simulink model "pt8612_dpll_fpga"  (Simulink 5.0)
settings: Solver=ode45  StartTime=0.0  StopTime=10  RelTol=1e-9  AbsTol=1e-12
values from neighbouring files (symbols this model uses):
  alpha = 2^-24    (= 5.96046447754e-08)    [DPLL_init_2.m]    (also in pt8612_dpll_fpga_init.m = -7; pt8612_dpll_fpga_init_2.m = -5)
  beta = 2^-10    (= 0.0009765625)    [DPLL_init_2.m]    (also in pt8612_dpll_fpga_init.m = 5; pt8612_dpll_fpga_init_2.m = 6)
  C = 680e-9    (= 6.8e-07)    [DPLL_init_2.m]    (also in pt8612_analog_pll_init.m = [1 0]; pt8612_analog_pll_init_2.m = [0 1 0]; pt8612_dpll_fpga_init.m; pt8612_dpll_fpga_init_2.m)
  fvcxo = 148.5e6/1.001    (= 148351648.352)    [DPLL_init_2.m]    (also in pt8612_analog_pll_init.m; pt8612_analog_pll_init_2.m; pt8612_dpll_fpga_init.m; pt8612_dpll_fpga_init_2.m = 148500000)
  Kvcxo = 90e-6    (= 9e-05)    [DPLL_init_2.m]    (also in pt8612_analog_pll_init.m; pt8612_analog_pll_init_2.m; pt8612_dpll_fpga_init.m; pt8612_dpll_fpga_init_2.m)
  Mdac = 3/4    (= 0.75)    [DPLL_init_2.m]    (also in pt8612_dpll_fpga_init.m = 1; pt8612_dpll_fpga_init_2.m = 1)
  Nbits = 16    [DPLL_init_2.m]    (also in pt8612_dpll_fpga_init.m; pt8612_dpll_fpga_init_2.m)
  Ndec1 = 91    [DPLL_init_2.m]    (also in pt8612_analog_pll_init.m; pt8612_analog_pll_init_2.m; pt8612_dpll_fpga_init.m = 364)
  Ndec2 = 500    [DPLL_init_2.m]    (also in pt8612_analog_pll_init.m; pt8612_analog_pll_init_2.m; pt8612_dpll_fpga_init.m = 2000)
  R = 1/(wkneeloop*20)/C    (= 4060.30501089)    [DPLL_init_2.m]    (also in pt8612_dpll_fpga_init.m; pt8612_dpll_fpga_init_2.m = 3900)
  Tdac = 4/148.5e6    (= 2.6936026936e-08)    [DPLL_init_2.m]    (also in pt8612_dpll_fpga_init.m)
  Tpll = 1/fpll    (= 3.37037037037e-06)    [DPLL_init_2.m]    (also in pt8612_dpll_fpga_init.m = 1.34814814815e-05)
  Vcc = 3.3    [DPLL_init_2.m]    (also in pt8612_analog_pll_init.m; pt8612_analog_pll_init_2.m; pt8612_dpll_fpga_init.m = 2.5; pt8612_dpll_fpga_init_2.m = 2.5)
  Vvcxo0 = 1.25    [DPLL_init_2.m]    (also in pt8612_analog_pll_init.m; pt8612_analog_pll_init_2.m; pt8612_dpll_fpga_init.m; pt8612_dpll_fpga_init_2.m)
  Vvcxomax = 2.5    [DPLL_init_2.m]    (also in pt8612_analog_pll_init.m; pt8612_analog_pll_init_2.m; pt8612_dpll_fpga_init.m; pt8612_dpll_fpga_init_2.m)
  Vvcxomin = 0    [DPLL_init_2.m]    (also in pt8612_analog_pll_init.m; pt8612_analog_pll_init_2.m; pt8612_dpll_fpga_init.m; pt8612_dpll_fpga_init_2.m)
libraries: simulink x3
settings Model: LastModifiedBy=thh

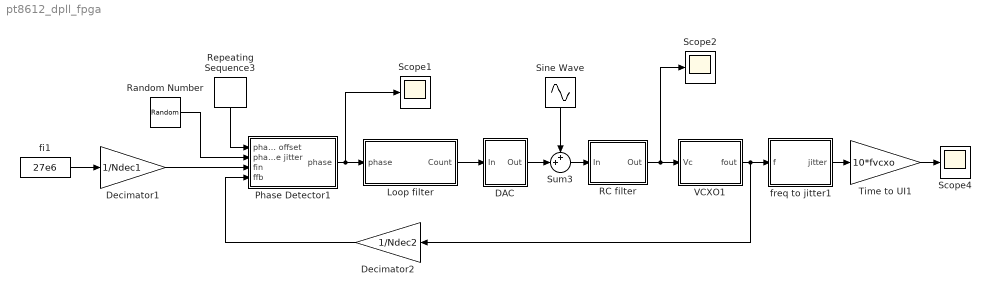
== system pt8612_dpll_fpga ==
  DAC : Subsystem
  Decimator1 : Gain  Gain=1/Ndec1  SaturateOnIntegerOverflow=on
  Decimator2 : Gain  Orientation=left  Gain=1/Ndec2  SaturateOnIntegerOverflow=on
  Loop filter : Subsystem
  Phase Detector1 : Subsystem
  RC filter : Subsystem
  Random Number : RandomNumber  Variance=0  SampleTime=Tpll
  Repeating Sequence3 : simulink/Sources/Repeating Sequence  Orientation=down  rep_seq_t=[0 0.5 0.5 1]*5  rep_seq_y=[0 0 1 1]*5
  Scope1 : Scope
      settings: TimeRange=10  YMin=-250  YMax=5500  SampleInput=on  SampleTime=Tpll
  Scope2 : Scope
      settings: TimeRange=10  YMin=0.22  YMax=0.29  SaveName=ScopeData3  SampleInput=on  SampleTime=1e-4
  Scope4 : Scope
      settings: TimeRange=10  YMin=-3020  YMax=-2977.5  SaveName=ScopeData2  SampleInput=on  SampleTime=1e-4
  Sine Wave : Sin  Orientation=down  Amplitude=0  Frequency=2*pi*25  SampleTime=0
  Sum3 : Sum  Inputs=++|  SaturateOnIntegerOverflow=on
  Time to UI1 : Gain  Gain=10*fvcxo  SaturateOnIntegerOverflow=on
  VCXO1 : Subsystem
  fi1 : Constant  Value=27e6
  freq to jitter1 : Subsystem
  wires:
  freq to jitter1/1(jitter) -> Time to UI1/1
  Time to UI1/1 -> Scope4/1
  Decimator2/1 -> Phase Detector1/4(ffb)
  Phase Detector1/1(phase) -> Loop filter/1(phase), Scope1/1
  Decimator1/1 -> Phase Detector1/3(fin)
  fi1/1 -> Decimator1/1
  RC filter/1(Out) -> VCXO1/1(Vc), Scope2/1
  Repeating Sequence3/1 -> Phase Detector1/1(phase offset)
  Random Number/1 -> Phase Detector1/2(phase jitter)
  DAC/1(Out) -> Sum3/2
  Sum3/1 -> RC filter/1(In)
  VCXO1/1(fout) -> freq to jitter1/1(f), Decimator2/1
  Loop filter/1(Count) -> DAC/1(In)
  Sine Wave/1 -> Sum3/1

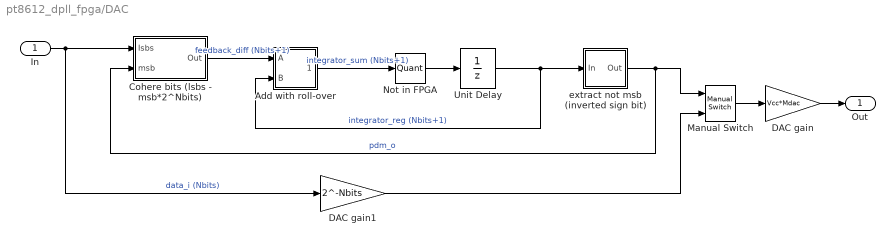
== system pt8612_dpll_fpga/DAC ==
  In : Inport
  Add with roll-over : Subsystem
  Cohere bits (lsbs - msb*2^Nbits) : Subsystem
  DAC gain : Gain  Gain=Vcc*Mdac  SaturateOnIntegerOverflow=on
  DAC gain1 : Gain  Gain=2^-Nbits  SaturateOnIntegerOverflow=on
  Manual Switch : simulink/Signal Routing/Manual Switch  sw=0  action=0
  Not in FPGA : Quantizer  QuantizationInterval=1
  Unit Delay : UnitDelay  SampleTime=Tdac
  extract not msb (inverted sign bit) : Subsystem
  Out : Outport
  wires:
  In/1 -> DAC gain1/1, Cohere bits (lsbs - msb*2^Nbits)/1(Isbs)  "data_i (Nbits)"
  extract not msb (inverted sign bit)/1(Out) -> Cohere bits (lsbs - msb*2^Nbits)/2(msb), Manual Switch/1  "pdm_o"
  Unit Delay/1 -> Add with roll-over/2(B), extract not msb (inverted sign bit)/1(In)  "integrator_reg (Nbits+1)"
  DAC gain/1 -> Out/1
  Not in FPGA/1 -> Unit Delay/1
  Cohere bits (lsbs - msb*2^Nbits)/1(Out) -> Add with roll-over/1(A)  "feedback_diff (Nbits+1)"
  Add with roll-over/1(A+B) -> Not in FPGA/1  "integrator_sum (Nbits+1)"
  DAC gain1/1 -> Manual Switch/2
  Manual Switch/1 -> DAC gain/1

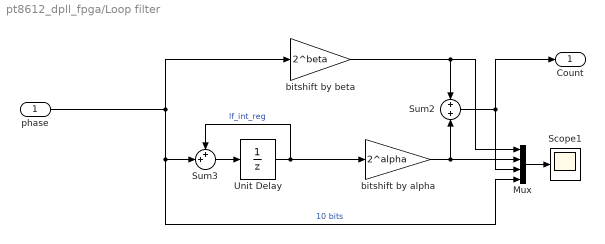
== system pt8612_dpll_fpga/Loop filter ==
  phase : Inport
  Mux : Mux
  Scope1 : Scope
      settings: TimeRange=10  YMin=-500  YMax=9000  SaveName=ScopeData5  Decimation=100  SampleInput=on  SampleTime=Tpll*100
  Sum2 : Sum  SaturateOnIntegerOverflow=on
  Sum3 : Sum  Inputs=++|  SaturateOnIntegerOverflow=on
  Unit Delay : UnitDelay  X0=3.31e4*2^9  SampleTime=Tpll
  bitshift by alpha : Gain  Gain=2^alpha  SaturateOnIntegerOverflow=on
  bitshift by beta : Gain  Gain=2^beta  SaturateOnIntegerOverflow=on
  Count : Outport
  wires:
  phase/1 -> bitshift by beta/1, Mux/4, Sum3/2  "10 bits"
  Sum2/1 -> Count/1, Mux/3
  bitshift by beta/1 -> Sum2/1, Mux/1
  bitshift by alpha/1 -> Sum2/2, Mux/2
  Mux/1 -> Scope1/1
  Unit Delay/1 -> bitshift by alpha/1, Sum3/1  "lf_int_reg"
  Sum3/1 -> Unit Delay/1

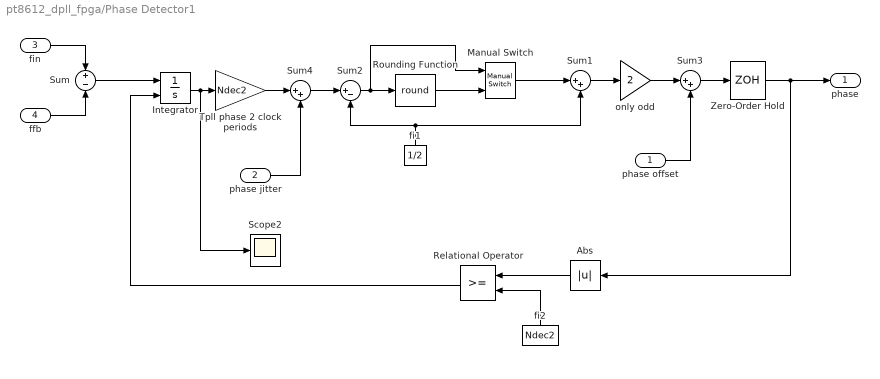
== system pt8612_dpll_fpga/Phase Detector1 ==
  phase offset : Inport
  phase jitter : Inport  Port=2
  fin : Inport  Port=3
  ffb : Inport  Port=4
  Abs : Abs  Orientation=left  SaturateOnIntegerOverflow=on
  Integrator : Integrator  ExternalReset=level
  Manual Switch : simulink/Signal Routing/Manual Switch  sw=0  action=0
  Relational Operator : RelationalOperator  Orientation=left
  Rounding Function : Rounding  Operator=round
  Scope2 : Scope
      settings: TimeRange=10  YMin=1.38778e-017  YMax=0.5  SampleInput=on  SampleTime=1e-4
  Sum : Sum  Inputs=+-  SaturateOnIntegerOverflow=on
  Sum1 : Sum  Inputs=|++  SaturateOnIntegerOverflow=on
  Sum2 : Sum  Inputs=|+-  SaturateOnIntegerOverflow=on
  Sum3 : Sum  Inputs=|++  SaturateOnIntegerOverflow=on
  Sum4 : Sum  Inputs=|++  SaturateOnIntegerOverflow=on
  Tpll phase 2 clock periods : Gain  Gain=Ndec2  SaturateOnIntegerOverflow=on
  Zero-Order Hold : ZeroOrderHold  SampleTime=Tpll
  fi1 : Constant  Orientation=up  Value=1/2
  fi2 : Constant  Orientation=up  Value=Ndec2
  only odd : Gain  Gain=2  SaturateOnIntegerOverflow=on
  phase : Outport
  wires:
  ffb/1 -> Sum/2
  fin/1 -> Sum/1
  Sum/1 -> Integrator/1
  Integrator/1 -> Tpll phase 2 clock periods/1, Scope2/1
  fi1/1 -> Sum1/2, Sum2/2
  Sum2/1 -> Manual Switch/1, Rounding Function/1
  phase offset/1 -> Sum3/2
  Sum3/1 -> Zero-Order Hold/1
  Sum1/1 -> only odd/1
  Manual Switch/1 -> Sum1/1
  Rounding Function/1 -> Manual Switch/2
  phase jitter/1 -> Sum4/2
  Sum4/1 -> Sum2/1
  Tpll phase 2 clock periods/1 -> Sum4/1
  only odd/1 -> Sum3/1
  Abs/1 -> Relational Operator/1
  fi2/1 -> Relational Operator/2
  Relational Operator/1 -> Integrator/2
  Zero-Order Hold/1 -> phase/1, Abs/1

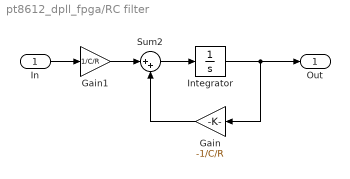
== system pt8612_dpll_fpga/RC filter ==
  In : Inport
  Gain : Gain  Orientation=left  Gain=-1/C/R  SaturateOnIntegerOverflow=on
  Gain1 : Gain  Gain=1/C/R  SaturateOnIntegerOverflow=on
  Integrator : Integrator  InitialCondition=Vvcxo0
  Sum2 : Sum  Inputs=|++  SaturateOnIntegerOverflow=on
  Out : Outport
  wires:
  In/1 -> Gain1/1
  Integrator/1 -> Out/1, Gain/1
  Sum2/1 -> Integrator/1
  Gain/1 -> Sum2/2
  Gain1/1 -> Sum2/1

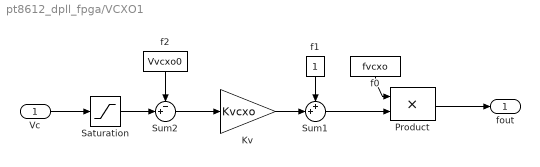
== system pt8612_dpll_fpga/VCXO1 ==
  Vc : Inport
  Kv : Gain  Gain=Kvcxo  SaturateOnIntegerOverflow=on
  Product : Product  SaturateOnIntegerOverflow=on
  Saturation : Saturate  UpperLimit=Vvcxomax  LowerLimit=Vvcxomin
  Sum1 : Sum  Inputs=++|  SaturateOnIntegerOverflow=on
  Sum2 : Sum  Inputs=-+|  SaturateOnIntegerOverflow=on
  f0 : Constant  Orientation=down  Value=fvcxo
  f1 : Constant  Orientation=down
  f2 : Constant  Orientation=down  Value=Vvcxo0
  fout : Outport
  wires:
  f2/1 -> Sum2/1
  Vc/1 -> Saturation/1
  Sum2/1 -> Kv/1
  Product/1 -> fout/1
  Kv/1 -> Sum1/2
  Sum1/1 -> Product/2
  f1/1 -> Sum1/1
  f0/1 -> Product/1
  Saturation/1 -> Sum2/2

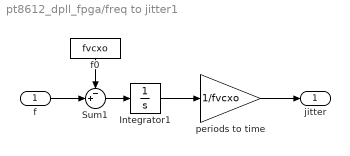
== system pt8612_dpll_fpga/freq to jitter1 ==
  f : Inport
  Integrator1 : Integrator
  Sum1 : Sum  Inputs=-+|  SaturateOnIntegerOverflow=on
  f0 : Constant  Orientation=down  Value=fvcxo
  periods to time : Gain  Gain=1/fvcxo  SaturateOnIntegerOverflow=on
  jitter : Outport
  wires:
  periods to time/1 -> jitter/1
  f/1 -> Sum1/2
  f0/1 -> Sum1/1
  Sum1/1 -> Integrator1/1
  Integrator1/1 -> periods to time/1

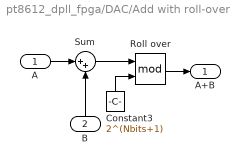
== system pt8612_dpll_fpga/DAC/Add with roll-over ==
  A : Inport
  B : Inport  Orientation=up  Port=2
  Constant3 : Constant  Orientation=up  Value=2^(Nbits+1)
  Roll over : Math  Operator=mod
  Sum : Sum  Inputs=|++  SaturateOnIntegerOverflow=on
  A+B : Outport
  wires:
  Sum/1 -> Roll over/1
  Constant3/1 -> Roll over/2
  B/1 -> Sum/2
  A/1 -> Sum/1
  Roll over/1 -> A+B/1

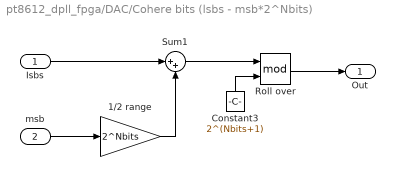
== system pt8612_dpll_fpga/DAC/Cohere bits (lsbs - msb*2^Nbits) ==
  Isbs : Inport
  msb : Inport  Port=2
  1/2 range : Gain  Gain=2^Nbits  SaturateOnIntegerOverflow=on
  Constant3 : Constant  Orientation=up  Value=2^(Nbits+1)
  Roll over : Math  Operator=mod
  Sum1 : Sum  Inputs=|++  SaturateOnIntegerOverflow=on
  Out : Outport
  wires:
  Sum1/1 -> Roll over/1
  1/2 range/1 -> Sum1/2
  Constant3/1 -> Roll over/2
  msb/1 -> 1/2 range/1
  Isbs/1 -> Sum1/1
  Roll over/1 -> Out/1

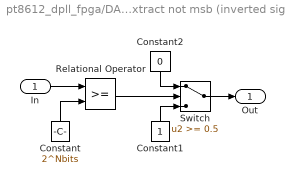
== system pt8612_dpll_fpga/DAC/extract not msb (inverted sign bit) ==
  In : Inport
  Constant : Constant  Orientation=up  Value=2^Nbits
  Constant1 : Constant  Orientation=up
  Constant2 : Constant  Orientation=down  Value=0
  Relational Operator : RelationalOperator
  Switch : Switch  Threshold=0.5  SaturateOnIntegerOverflow=on
  Out : Outport
  wires:
  Constant/1 -> Relational Operator/2
  In/1 -> Relational Operator/1
  Relational Operator/1 -> Switch/2
  Constant2/1 -> Switch/1
  Constant1/1 -> Switch/3
  Switch/1 -> Out/1
